simulink model "dianrong_KF"  (R2023b)
settings: Solver=VariableStepAuto  StartTime=0.0  StopTime=10.0  RelTol=1e-3
settings Model: Creator=CSC  LastModifiedBy=CSC

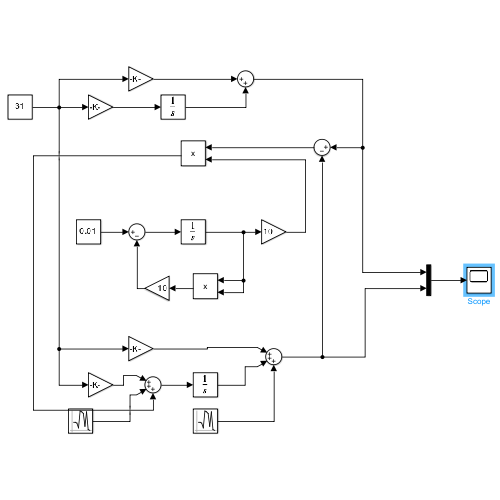
[thumbnail: Simulink's stored preview of the top-level diagram]
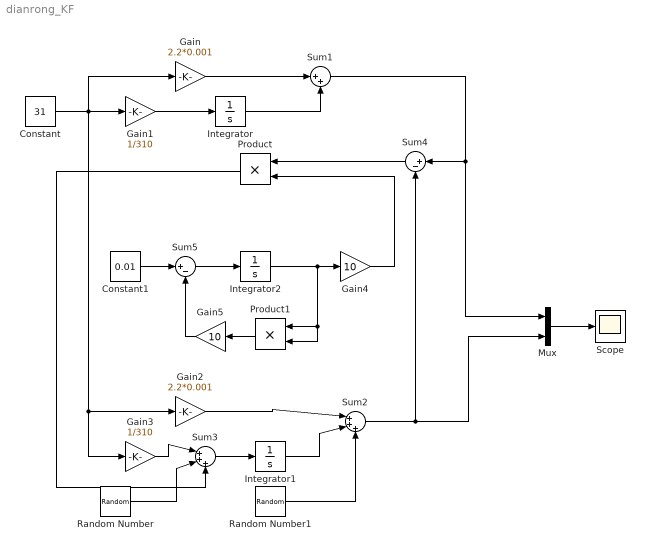
== system dianrong_KF ==
  Constant : Constant  Value=31
  Constant1 : Constant  Value=0.01
  Gain : Gain  Gain=2.2*0.001
  Gain1 : Gain  Gain=1/310
  Gain2 : Gain  Gain=2.2*0.001
  Gain3 : Gain  Gain=1/310
  Gain4 : Gain  Gain=10
  Gain5 : Gain  Gain=10
  Integrator : Integrator
  Integrator1 : Integrator
  Integrator2 : Integrator
  Mux : Mux  Inputs=2
  Product : Product
  Product1 : Product
  Random Number : RandomNumber  Variance=0.01  SampleTime=0.1
  Random Number1 : RandomNumber  Variance=0.1  SampleTime=0.1
  Scope : Scope
  Sum1 : Sum  Inputs=|++
  Sum2 : Sum  Inputs=|+++
  Sum3 : Sum  Inputs=|+++
  Sum4 : Sum  Inputs=|+-
  Sum5 : Sum  Inputs=|+-
  wires:
  Sum1/1 -> Mux/1, Sum4/1
  Gain/1 -> Sum1/1
  Integrator/1 -> Sum1/2
  Gain1/1 -> Integrator/1
  Gain2/1 -> Sum2/1
  Constant/1 -> Gain3/1, Gain2/1, Gain1/1, Gain/1
  Integrator1/1 -> Sum2/2
  Random Number/1 -> Sum3/2
  Gain3/1 -> Sum3/1
  Sum3/1 -> Integrator1/1
  Random Number1/1 -> Sum2/3
  Sum2/1 -> Sum4/2, Mux/2
  Sum4/1 -> Product/1
  Integrator2/1 -> Product1/1, Product1/2, Gain4/1
  Gain4/1 -> Product/2
  Sum5/1 -> Integrator2/1
  Constant1/1 -> Sum5/1
  Product1/1 -> Gain5/1
  Gain5/1 -> Sum5/2
  Product/1 -> Sum3/3
  Mux/1 -> Scope/1
